simulink model "Problem_1_Part_F"  (R2018b)
settings: Solver=FixedStepAuto  StartTime=0.0  StopTime=10  FixedStep=0.0001  RelTol=1e-3
InitFcn:
  | Initial_Data
values from neighbouring files (symbols this model uses):
  e_max = 5:1:20    [emax_Variable_Part_F.m]
undefined symbols (not defined in the file or in its folder): aty, atz, g, G_p, Psi_m0, ro, S, T, T_1, T_2, Theta_m0, V_m0I
libraries: vrlib x2, simulink x1
settings Model: Creator=User  LastModifiedBy=User

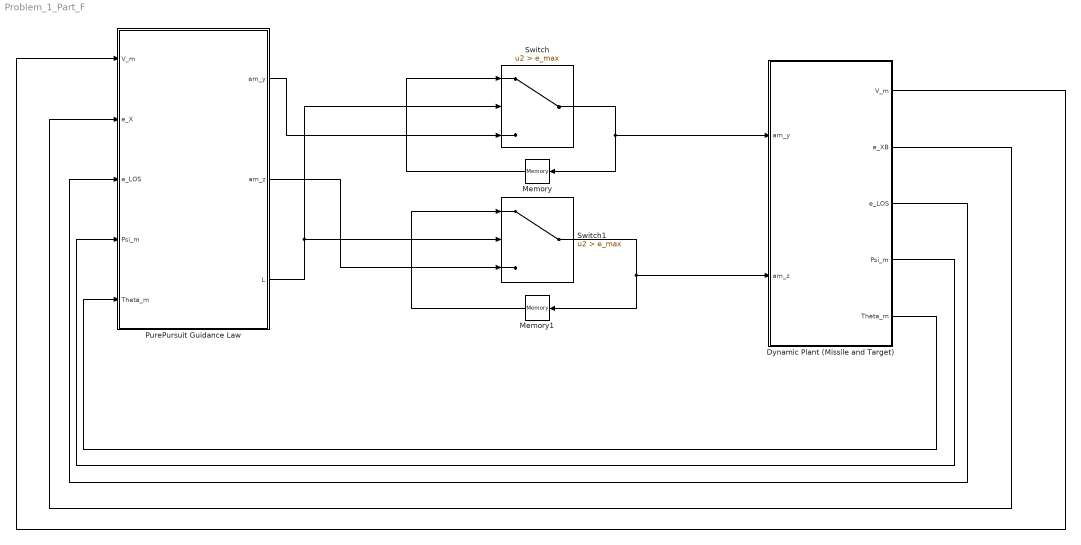
== system Problem_1_Part_F ==
  " PurePursuit Guidance Law" : Subsystem
  Dynamic Plant (Missile and Target) : Subsystem
  Memory : Memory
  Memory1 : Memory
  Switch : Switch  Criteria=u2 > Threshold  Threshold=e_max
  Switch1 : Switch  Criteria=u2 > Threshold  Threshold=e_max
  wires:
  Dynamic Plant (Missile and Target)/1(V_m) -> " PurePursuit Guidance Law"/1(V_m)
  Dynamic Plant (Missile and Target)/3(e_LOS) -> " PurePursuit Guidance Law"/3(e_LOS)
  Dynamic Plant (Missile and Target)/2(e_XB) -> " PurePursuit Guidance Law"/2(e_X)
  Switch/1 -> Dynamic Plant (Missile and Target)/1(am_y), Memory/1
  Dynamic Plant (Missile and Target)/5(Theta_m) -> " PurePursuit Guidance Law"/5(Theta_m)
  Switch1/1 -> Memory1/1, Dynamic Plant (Missile and Target)/2(am_z)
  Dynamic Plant (Missile and Target)/4(Psi_m) -> " PurePursuit Guidance Law"/4(Psi_m)
  Memory1/1 -> Switch1/1
  " PurePursuit Guidance Law"/2(am_z) -> Switch1/3
  " PurePursuit Guidance Law"/3(L) -> Switch1/2, Switch/2
  Memory/1 -> Switch/1
  " PurePursuit Guidance Law"/1(am_y) -> Switch/3

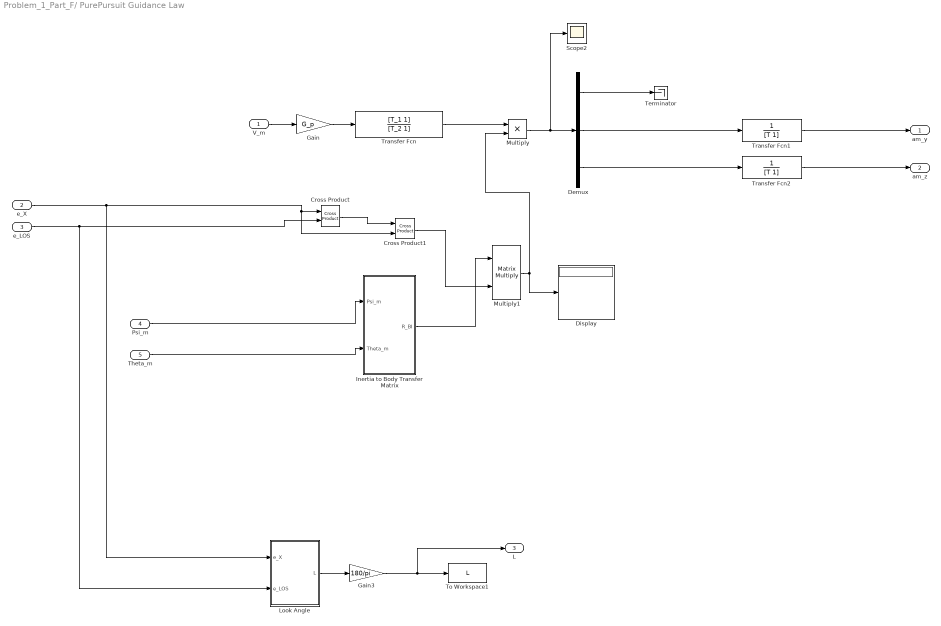
== system Problem_1_Part_F/ PurePursuit Guidance Law ==
  V_m : Inport
  e_X : Inport  Port=2
  e_LOS : Inport  Port=3
  Psi_m : Inport  Port=4
  Theta_m : Inport  Port=5
  Cross Product : vrlib/Utilities/Cross Product
      settings: SourceProductBaseCode=VR
  Cross Product1 : vrlib/Utilities/Cross Product
      settings: SourceProductBaseCode=VR
  Demux : Demux  Outputs=3
  Display : Display
  Gain : Gain  Gain=G_p
  Gain3 : Gain  Gain=180/pi
  Inertia to Body Transfer Matrix : MATLAB Function  TreatAsAtomicUnit=on
  Look Angle : MATLAB Function  TreatAsAtomicUnit=on
  Multiply : Product
  Multiply1 : Product  Multiplication=Matrix(*)
  Scope2 : Scope
  Terminator : Terminator
  To Workspace1 : ToWorkspace  VariableName=L  SaveFormat=Timeseries  SampleTime=-1
  Transfer Fcn : TransferFcn  Numerator=[T_1 1]  Denominator=[T_2 1]
  Transfer Fcn1 : TransferFcn  Denominator=[T 1]
  Transfer Fcn2 : TransferFcn  Denominator=[T 1]
  am_y : Outport
  am_z : Outport  Port=2
  L : Outport  Port=3
  wires:
  Demux/2 -> Transfer Fcn1/1
  Gain/1 -> Transfer Fcn/1
  V_m/1 -> Gain/1
  Transfer Fcn/1 -> Multiply/1
  Cross Product/1 -> Cross Product1/1
  Multiply/1 -> Scope2/1, Demux/1
  Demux/1 -> Terminator/1
  Demux/3 -> Transfer Fcn2/1
  Transfer Fcn1/1 -> am_y/1
  Transfer Fcn2/1 -> am_z/1
  Psi_m/1 -> Inertia to Body Transfer Matrix/1(Psi_m)
  Theta_m/1 -> Inertia to Body Transfer Matrix/2(Theta_m)
  Inertia to Body Transfer Matrix/1(R_BI) -> Multiply1/1
  Cross Product1/1 -> Multiply1/2
  Multiply1/1 -> Display/1, Multiply/2
  Look Angle/1(L) -> Gain3/1
  e_X/1 -> Look Angle/1(e_X), Cross Product/1, Cross Product1/2
  e_LOS/1 -> Look Angle/2(e_LOS), Cross Product/2
  Gain3/1 -> L/1, To Workspace1/1

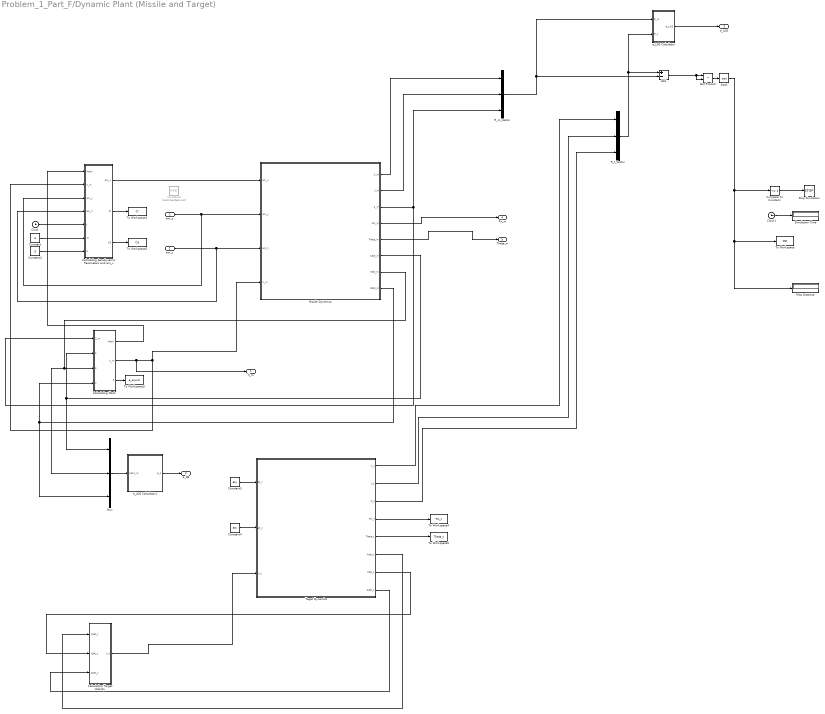
== system Problem_1_Part_F/Dynamic Plant (Missile and Target) ==
  am_y : Inport
  am_z : Inport  Port=2
  Add : Sum  Inputs=+-
  Calculating Aerodynamic Parameters and am_x : MATLAB Function  TreatAsAtomicUnit=on
  Calculating Mach : MATLAB Function  TreatAsAtomicUnit=on
  Calculating Target Velocity : MATLAB Function  TreatAsAtomicUnit=on
  Clock : Clock
  Clock1 : Clock
  Compare To Constant : simulink/Logic and Bit Operations/Compare To Constant  relop=<=  const=4  OutDataTypeStr=boolean
  Constant : Constant  Value=ro
  Constant1 : Constant  Value=S
  Constant2 : Constant  Commented=on  Value=4*9.81
  Constant3 : Constant  Value=aty
  Constant4 : Constant  Value=atz
  Dot Product : DotProduct  InputSameDT=on  OutDataTypeStr=Inherit: Inherit via internal rule
  Miss Distance : Display
  Missile Dynamics : Subsystem
  Mux : Mux  Inputs=3
  R_m_Vector : Mux  Inputs=3
  R_t_Vector : Mux  Inputs=3
  Simulation Time : Display
  Sqrt1 : Sqrt  SaturateOnIntegerOverflow=on
  Stop Simulation : Stop
  Taget Dynamics : Subsystem
  To Workspace : ToWorkspace  VariableName=MD  SampleTime=-1
  To Workspace1 : ToWorkspace  VariableName=Cl  SaveFormat=Timeseries  SampleTime=-1
  To Workspace2 : ToWorkspace  VariableName=Cd  SaveFormat=Timeseries  SampleTime=-1
  To Workspace3 : ToWorkspace  VariableName=a_sound  SaveFormat=Timeseries  SampleTime=-1
  To Workspace4 : ToWorkspace  VariableName=Psi_t  SaveFormat=Timeseries  SampleTime=-1
  To Workspace5 : ToWorkspace  VariableName=Theta_t  SaveFormat=Timeseries  SampleTime=-1
  e_LOS Calculator : MATLAB Function  TreatAsAtomicUnit=on
  e_LOS Calculator1 : MATLAB Function  TreatAsAtomicUnit=on
  V_m : Outport
  e_XB : Outport  Port=2
  e_LOS : Outport  Port=3
  Psi_m : Outport  Port=4
  Theta_m : Outport  Port=5
  wires:
  Taget Dynamics/6(Xdot_t) -> Calculating Target Velocity/1(Xdot_t)
  Taget Dynamics/3(Z_t) -> R_t_Vector/3
  am_y/1 -> Calculating Aerodynamic Parameters and am_x/3(am_y), Missile Dynamics/2(am_y)
  Missile Dynamics/2(Y_m) -> R_m_Vector/2
  Calculating Target Velocity/1(V_t) -> Taget Dynamics/3(V_t)
  Missile Dynamics/3(Z_m) -> Calculating Mach/1(Z_m), R_m_Vector/3
  Missile Dynamics/1(X_m) -> R_m_Vector/1
  Clock/1 -> Calculating Aerodynamic Parameters and am_x/5(t)
  am_z/1 -> Calculating Aerodynamic Parameters and am_x/4(am_z), Missile Dynamics/3(am_z)
  Missile Dynamics/8(Zdot_m) -> Mux/3, Calculating Mach/4(Zdot_m)
  Constant/1 -> Calculating Aerodynamic Parameters and am_x/6(ro)
  Calculating Mach/1(Mach) -> Calculating Aerodynamic Parameters and am_x/1(Mach)
  Taget Dynamics/1(X_t) -> R_t_Vector/1
  Missile Dynamics/6(Xdot_m) -> Mux/1, Calculating Mach/2(Xdot_m)
  Constant1/1 -> Calculating Aerodynamic Parameters and am_x/7(S)
  Taget Dynamics/7(Ydot_t) -> Calculating Target Velocity/2(Ydot_t)
  Missile Dynamics/7(Ydot_m) -> Calculating Mach/3(Ydot_m), Mux/2
  Missile Dynamics/4(Psi_m) -> Psi_m/1
  Calculating Aerodynamic Parameters and am_x/1(am_x) -> Missile Dynamics/1(am_x)
  Taget Dynamics/2(Y_t) -> R_t_Vector/2
  Calculating Mach/2(V_m) -> V_m/1, Calculating Aerodynamic Parameters and am_x/2(V_m), Missile Dynamics/4(V_m)
  Missile Dynamics/5(Theta_m) -> Theta_m/1
  Constant3/1 -> Taget Dynamics/1(at_y)
  Constant4/1 -> Taget Dynamics/2(at_z)
  Taget Dynamics/8(Zdot_t) -> Calculating Target Velocity/3(Zdot_t)
  Dot Product/1 -> Sqrt1/1
  Clock1/1 -> Simulation Time/1
  R_m_Vector/1 -> e_LOS Calculator/1(R_m), Add/2
  Add/1 -> Dot Product/2, Dot Product/1
  R_t_Vector/1 -> e_LOS Calculator/2(R_t), Add/1
  e_LOS Calculator/1(e_LOS) -> e_LOS/1
  e_LOS Calculator1/1(e_X) -> e_XB/1
  Mux/1 -> e_LOS Calculator1/1(VecV_m)
  Sqrt1/1 -> Miss Distance/1, To Workspace/1, Compare To Constant/1
  Compare To Constant/1 -> Stop Simulation/1
  Calculating Aerodynamic Parameters and am_x/2(Cl) -> To Workspace1/1
  Calculating Aerodynamic Parameters and am_x/3(Cd) -> To Workspace2/1
  Calculating Mach/3(a_sound) -> To Workspace3/1
  Taget Dynamics/4(Psi_t) -> To Workspace4/1
  Taget Dynamics/5(Theta_t) -> To Workspace5/1

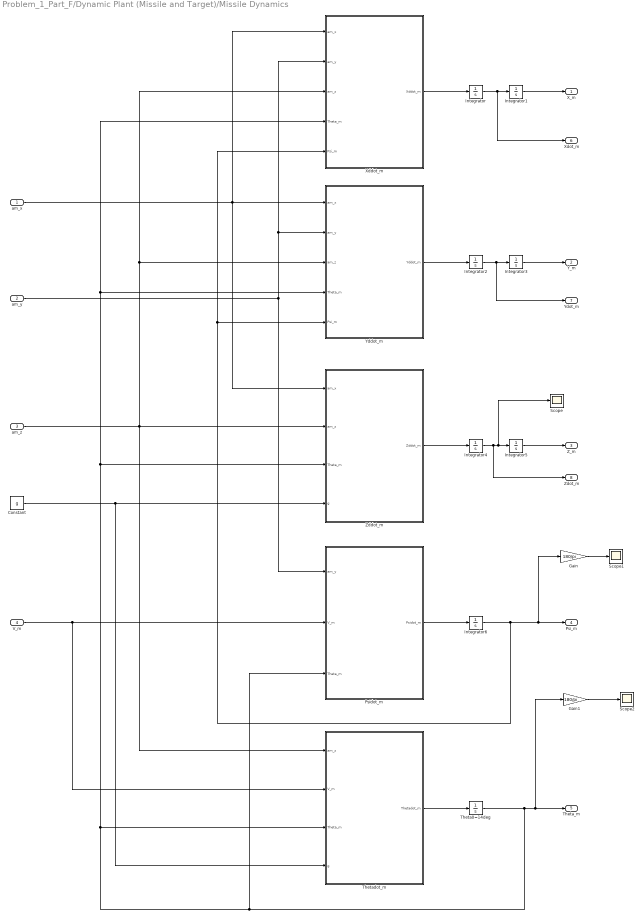
== system Problem_1_Part_F/Dynamic Plant (Missile and Target)/Missile Dynamics ==
  am_x : Inport
  am_y : Inport  Port=2
  am_z : Inport  Port=3
  V_m : Inport  Port=4
  Constant : Constant  Value=g
  Gain : Gain  Gain=180/pi
  Gain1 : Gain  Gain=180/pi
  Integrator : Integrator  InitialCondition=V_m0I(1)
  Integrator1 : Integrator  InitialCondition=0.001
  Integrator2 : Integrator  InitialCondition=V_m0I(2)
  Integrator3 : Integrator
  Integrator4 : Integrator  InitialCondition=V_m0I(3)
  Integrator5 : Integrator
  Integrator6 : Integrator  InitialCondition=Psi_m0
  Psidot_m : MATLAB Function  TreatAsAtomicUnit=on
  Scope : Scope
  Scope1 : Scope
  Scope2 : Scope
  Theta0=14deg : Integrator  InitialCondition=Theta_m0
  Thetadot_m : MATLAB Function  TreatAsAtomicUnit=on
  Xddot_m : MATLAB Function  TreatAsAtomicUnit=on
  Yddot_m : MATLAB Function  TreatAsAtomicUnit=on
  Zddot_m : MATLAB Function  TreatAsAtomicUnit=on
  X_m : Outport
  Y_m : Outport  Port=2
  Z_m : Outport  Port=3
  Psi_m : Outport  Port=4
  Theta_m : Outport  Port=5
  Xdot_m : Outport  Port=6
  Ydot_m : Outport  Port=7
  Zdot_m : Outport  Port=8
  wires:
  am_x/1 -> Yddot_m/1(am_x), Xddot_m/1(am_x), Zddot_m/1(am_x)
  am_y/1 -> Psidot_m/1(am_y), Xddot_m/2(am_y), Yddot_m/2(am_y)
  am_z/1 -> Xddot_m/3(am_z), Yddot_m/3(am_z), Zddot_m/2(am_z), Thetadot_m/1(am_z)
  Xddot_m/1(Xddot_m) -> Integrator/1
  Integrator/1 -> Integrator1/1, Xdot_m/1
  Integrator1/1 -> X_m/1
  Integrator3/1 -> Y_m/1
  Yddot_m/1(Yddot_m) -> Integrator2/1
  Zddot_m/1(Zddot_m) -> Integrator4/1
  Constant/1 -> Zddot_m/4(g), Thetadot_m/4(g)
  Psidot_m/1(Psidot_m) -> Integrator6/1
  Integrator6/1 -> Gain/1, Psi_m/1, Xddot_m/5(Psi_m), Yddot_m/5(Psi_m)
  Thetadot_m/1(Thetadot_m) -> Theta0=14deg/1
  Theta0=14deg/1 -> Psidot_m/3(Theta_m), Thetadot_m/3(Theta_m), Zddot_m/3(Theta_m), Yddot_m/4(Theta_m), Xddot_m/4(Theta_m), Gain1/1, Theta_m/1
  Integrator5/1 -> Z_m/1
  Integrator4/1 -> Scope/1, Integrator5/1, Zdot_m/1
  Integrator2/1 -> Ydot_m/1, Integrator3/1
  V_m/1 -> Psidot_m/2(V_m), Thetadot_m/2(V_m)
  Gain/1 -> Scope1/1
  Gain1/1 -> Scope2/1

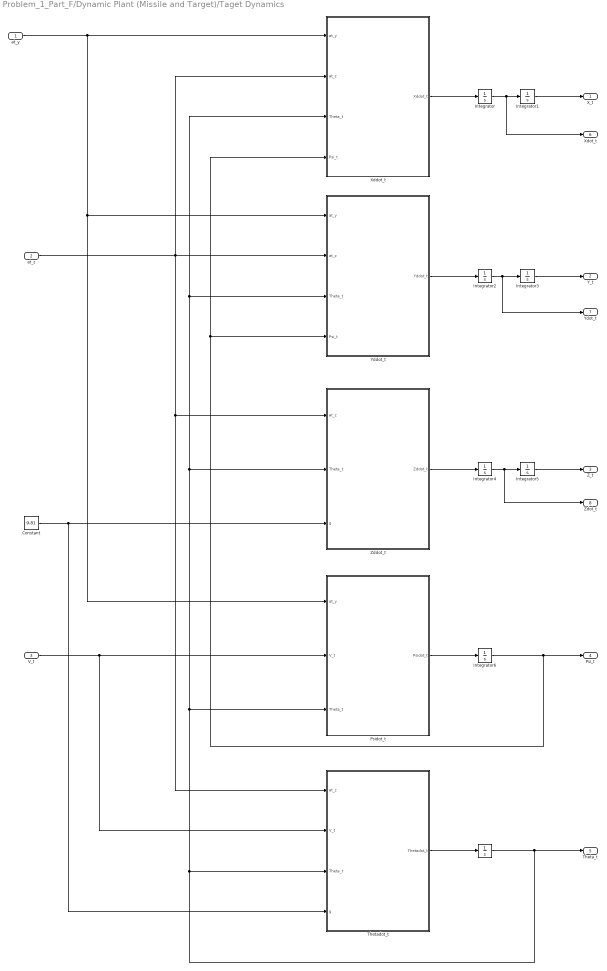
== system Problem_1_Part_F/Dynamic Plant (Missile and Target)/Taget Dynamics ==
  at_y : Inport
  at_z : Inport  Port=2
  V_t : Inport  Port=3
  " " : Integrator
  Constant : Constant  Value=9.81
  Integrator : Integrator  InitialCondition=-300
  Integrator1 : Integrator  InitialCondition=12000
  Integrator2 : Integrator
  Integrator3 : Integrator
  Integrator4 : Integrator
  Integrator5 : Integrator  InitialCondition=3000
  Integrator6 : Integrator  InitialCondition=3.14159
  Psidot_t : MATLAB Function  TreatAsAtomicUnit=on
  Thetadot_t : MATLAB Function  TreatAsAtomicUnit=on
  Xddot_t : MATLAB Function  TreatAsAtomicUnit=on
  Yddot_t : MATLAB Function  TreatAsAtomicUnit=on
  Zddot_t : MATLAB Function  TreatAsAtomicUnit=on
  X_t : Outport
  Y_t : Outport  Port=2
  Z_t : Outport  Port=3
  Psi_t : Outport  Port=4
  Theta_t : Outport  Port=5
  Xdot_t : Outport  Port=6
  Ydot_t : Outport  Port=7
  Zdot_t : Outport  Port=8
  wires:
  Psidot_t/1(Psidot_t) -> Integrator6/1
  Integrator4/1 -> Zdot_t/1, Integrator5/1
  Xddot_t/1(Xddot_t) -> Integrator/1
  Thetadot_t/1(Thetadot_t) -> " "/1
  Yddot_t/1(Yddot_t) -> Integrator2/1
  Integrator2/1 -> Ydot_t/1, Integrator3/1
  Integrator/1 -> Integrator1/1, Xdot_t/1
  Zddot_t/1(Zddot_t) -> Integrator4/1
  at_y/1 -> Xddot_t/1(at_y), Yddot_t/1(at_y), Psidot_t/1(at_y)
  at_z/1 -> Yddot_t/2(at_z), Zddot_t/1(at_z), Thetadot_t/1(at_z), Xddot_t/2(at_z)
  Integrator1/1 -> X_t/1
  Integrator3/1 -> Y_t/1
  Integrator5/1 -> Z_t/1
  Integrator6/1 -> Yddot_t/4(Psi_t), Xddot_t/4(Psi_t), Psi_t/1
  " "/1 -> Thetadot_t/3(Theta_t), Psidot_t/3(Theta_t), Zddot_t/2(Theta_t), Yddot_t/3(Theta_t), Xddot_t/3(Theta_t), Theta_t/1
  Constant/1 -> Zddot_t/3(g), Thetadot_t/4(g)
  V_t/1 -> Psidot_t/2(V_t), Thetadot_t/2(V_t)

== matlab function Problem_1_Part_F/Dynamic Plant (Missile and Target)/Calculating Mach ==
  data: Mach output; Z_m input; Xdot_m input; V_m output; Ydot_m input; Zdot_m input; a_sound output
function [Mach,V_m,a_sound]  = fcn(Z_m,Xdot_m,Ydot_m,Zdot_m)

T = 290 - 0.0065*Z_m; %Temperature as a function of altitude%
gamma = 1.4; %Ratio of specific heats%
R = 286; %Gas Constant%
a_sound = sqrt(gamma*R*T);
V_m = sqrt((Xdot_m)^2 + (Ydot_m)^2 + (Zdot_m)^2);
Mach = V_m/a_sound;

== matlab function Problem_1_Part_F/Dynamic Plant (Missile and Target)/Calculating Aerodynamic Parameters and am_x ==
  data: Mach input; am_x output; V_m input; am_y input; am_z input; t input; Cl output; Cd output; ro input; S input
function [am_x,Cl,Cd] = fcn(Mach,V_m,am_y,am_z,t,ro,S)

% T=Thrust(N),m=Mass(kg)
if t < 4
    T = 80000;
elseif t < 23
    T = 15000;
else
    T = 0;
end

if t < 4
    m = 600;
elseif t < 20
    m = 400;
else
    m = 300;
end

if Mach < 0.8
    Cd0 = 0.5;
    K = 0.04;
elseif Mach < 1.2
    Cd0 = 0.4;
    K = 0.025;
elseif Mach < 2
    Cd0 = 0.7;
    K = 0.035;
elseif Mach < 3
    Cd0 = 0.55;
    K = 0.04;
else
    Cd0 = 0.475;
    K = 0.04;
end
Cl = (2*m*((am_y^2) + (am_z^2))^0.5)/(ro*(V_m^2)*S);
Cd = Cd0 + K*(Cl^2);
D = 0.5*Cd*ro*S*V_m^2;
am_x = (T-D)/m;

== matlab function Problem_1_Part_F/Dynamic Plant (Missile and Target)/Missile Dynamics/Xddot_m ==
  data: am_x input; Xddot_m output; am_y input; am_z input; Theta_m input; Psi_m input
function Xddot_m  = fcn(am_x,am_y,am_z,Theta_m,Psi_m)

Xddot_m = am_x*cos(Theta_m)*cos(Psi_m) - am_y*sin(Psi_m) - am_z*sin(Theta_m)*cos(Psi_m);

== matlab function Problem_1_Part_F/Dynamic Plant (Missile and Target)/Calculating Target Velocity ==
  data: V_t output; Xdot_t input; Ydot_t input; Zdot_t input
function V_t   = fcn(Xdot_t,Ydot_t,Zdot_t)

V_t = sqrt((Xdot_t)^2 + (Ydot_t)^2 + (Zdot_t)^2);

== matlab function Problem_1_Part_F/Dynamic Plant (Missile and Target)/Missile Dynamics/Yddot_m ==
  data: am_x input; Yddot_m output; am_y input; am_z input; Theta_m input; Psi_m input
function Yddot_m  = fcn(am_x,am_y,am_z,Theta_m,Psi_m)

Yddot_m = am_x*cos(Theta_m)*sin(Psi_m) + am_y*cos(Psi_m) - am_z*sin(Theta_m)*sin(Psi_m);

== matlab function Problem_1_Part_F/Dynamic Plant (Missile and Target)/Missile Dynamics/Zddot_m ==
  data: am_x input; Zddot_m output; am_z input; Theta_m input; g input
function Zddot_m  = fcn(am_x,am_z,Theta_m,g)

Zddot_m = am_x*sin(Theta_m) + am_z*cos(Theta_m) - g;

== matlab function Problem_1_Part_F/Dynamic Plant (Missile and Target)/Missile Dynamics/Psidot_m ==
  data: am_y input; Psidot_m output; V_m input; Theta_m input
function Psidot_m  = fcn(am_y,V_m,Theta_m)

Psidot_m = am_y/(V_m*cos(Theta_m));

== matlab function Problem_1_Part_F/Dynamic Plant (Missile and Target)/Missile Dynamics/Thetadot_m ==
  data: am_z input; Thetadot_m output; V_m input; Theta_m input; g input
function Thetadot_m  = fcn(am_z,V_m,Theta_m,g)

Thetadot_m = (am_z - g*cos(Theta_m))/(V_m);

== matlab function Problem_1_Part_F/Dynamic Plant (Missile and Target)/Taget Dynamics/Psidot_t ==
  data: at_y input; Psidot_t output; V_t input; Theta_t input
function Psidot_t  = fcn(at_y,V_t,Theta_t)

Psidot_t = at_y/(V_t*cos(Theta_t));

== matlab function Problem_1_Part_F/Dynamic Plant (Missile and Target)/Taget Dynamics/Thetadot_t ==
  data: at_z input; Thetadot_t output; V_t input; Theta_t input; g input
function Thetadot_t  = fcn(at_z,V_t,Theta_t,g)

Thetadot_t = (at_z - g*cos(Theta_t))/(V_t);

== matlab function Problem_1_Part_F/Dynamic Plant (Missile and Target)/Taget Dynamics/Xddot_t ==
  data: at_y input; Xddot_t output; at_z input; Theta_t input; Psi_t input
function Xddot_t  = fcn(at_y,at_z,Theta_t,Psi_t)

Xddot_t = -at_y*sin(Psi_t) - at_z*sin(Theta_t)*cos(Psi_t);

== matlab function Problem_1_Part_F/Dynamic Plant (Missile and Target)/Taget Dynamics/Yddot_t ==
  data: at_y input; Yddot_t output; at_z input; Theta_t input; Psi_t input
function Yddot_t  = fcn(at_y,at_z,Theta_t,Psi_t)

Yddot_t = at_y*cos(Psi_t) - at_z*sin(Theta_t)*sin(Psi_t);

== matlab function Problem_1_Part_F/Dynamic Plant (Missile and Target)/Taget Dynamics/Zddot_t ==
  data: at_z input; Zddot_t output; Theta_t input; g input
function Zddot_t  = fcn(at_z,Theta_t,g)

Zddot_t = at_z*cos(Theta_t) - g;

== matlab function Problem_1_Part_F/ PurePursuit Guidance Law/Inertia to Body Transfer Matrix ==
  data: R_BI output; Psi_m input; Theta_m input
function R_BI = fcn(Psi_m,Theta_m)

R_Psi = [cos(Psi_m) sin(Psi_m) 0;-sin(Psi_m) cos(Psi_m) 0;0 0 1];
R_Theta = [cos(Theta_m) 0 -sin(Theta_m);0 1 0;sin(Theta_m) 0 cos(Theta_m)];
R_BI = R_Theta*R_Psi;

== matlab function Problem_1_Part_F/ PurePursuit Guidance Law/Look Angle ==
  data: e_X input; L output; e_LOS input
function L  = fcn(e_X,e_LOS)

L = acos((dot(e_X,e_LOS))/(norm(e_X)*norm(e_LOS)));

== matlab function Problem_1_Part_F/Dynamic Plant (Missile and Target)/e_LOS Calculator ==
  data: R_m input; e_LOS output; R_t input
function e_LOS  = fcn(R_m,R_t)
e_LOS = (R_t-R_m)/(norm(R_t-R_m));

== matlab function Problem_1_Part_F/Dynamic Plant (Missile and Target)/e_LOS Calculator1 ==
  data: VecV_m input; e_X output
function e_X  = fcn(VecV_m)
e_X = (VecV_m)/(norm(VecV_m));
